simulink model "mainV02_28"  (R2016b)
settings: Solver=VariableStepAuto  StartTime=0.0  StopTime=Inf  FixedStep=0.001  MaxStep=0.2  RelTol=1e-2
undefined symbols (not defined in the file): checks, deltae_degrees, deltafl_degrees, deltafr_degrees, deltar_degrees, deltat_1, deltat_2, deltat_3, deltat_4, deltat_5, Earth, F, ft, groundReaction, initialValues, LD, Light, m, MIL, Newton, Raphson, s, sigbuilder_block, WGS84
libraries: aerolibutil x19, simulink x10, aerolibtransform2 x6, aerolibasang x4, aerolib6dofsys x4, aerolib6dof2 x4, aerolibwind2 x3, aerolibbdyn x3, aerolibconvert2 x3, aerolibconvert x2, vrlib x2, aerolibatmos2 x1
(part 5 of 5)

== system mainV02_28/LIBIS Plant/Propulsion/Variant_Motor_4/noMappedMotor_4/Propeller_4 ==
  RPM : Inport
  V_flight : Inport  Port=2
  airDensity : Inport  Port=3
  Constant : Constant  Value=5
  Constant1 : Constant  Value=3
  Constant2 : Constant  Value=4
  Constant3 : Constant  Value=2
  Cp Interpolation Using Prelookup : Interpolation_n-D  Table=LD.Propulsion.propeller4.Cp  ExtrapMethod=Clip  ValidIndexMayReachLast=on  InternalRulePriority=Speed
  Ct Interpolation Using Prelookup2 : Interpolation_n-D  Table=LD.Propulsion.propeller4.Ct  ExtrapMethod=Clip  ValidIndexMayReachLast=on  InternalRulePriority=Speed
  Diameter : Constant  Value=LD.Propulsion.propeller4.Diameter
  Gain : Gain  Gain=1/60
  Math Function{,1..3} (4 alike) : Math  Operator=pow  SaturateOnIntegerOverflow=on
  Prelookup4 : PreLookup  BreakpointsData=LD.Propulsion.propeller4.RPM  IndexSearchMethod=Evenly spaced points  UseLastBreakpoint=on
  Prelookup5 : PreLookup  BreakpointsData=LD.Propulsion.propeller4.V  UseLastBreakpoint=on
  Product : Product  Inputs=4
  Product1 : Product  Inputs=4
  RPM1 : InportShadow
  P_needed : Outport
  Thrust : Outport  Port=2
  wires:
  Diameter/1 -> Math Function2/1, Math Function/1  "D"
  Constant/1 -> Math Function/2  "5"
  Constant1/1 -> Math Function1/2  "3"
  Cp Interpolation Using Prelookup/1 -> Product/4  "Cp"
  Math Function1/1 -> Product/3  "n^3"
  Math Function/1 -> Product/2  "D^5"
  airDensity/1 -> Product/1, Product1/4  "airDensity"
  Product/1 -> P_needed/1  "Pneeded"
  Product1/1 -> Thrust/1  "Thrust"
  V_flight/1 -> Prelookup5/1  "V_flight"
  Constant2/1 -> Math Function2/2  "4"
  Math Function2/1 -> Product1/3  "D^4"
  Prelookup4/1 -> Cp Interpolation Using Prelookup/1, Ct Interpolation Using Prelookup2/1
  Prelookup4/2 -> Ct Interpolation Using Prelookup2/2, Cp Interpolation Using Prelookup/2
  Prelookup5/1 -> Cp Interpolation Using Prelookup/3, Ct Interpolation Using Prelookup2/3
  Prelookup5/2 -> Ct Interpolation Using Prelookup2/4, Cp Interpolation Using Prelookup/4
  Ct Interpolation Using Prelookup2/1 -> Product1/1  "Ct"
  Constant3/1 -> Math Function3/2  "2"
  Gain/1 -> Math Function1/1, Math Function3/1  "n_rev_s"
  Math Function3/1 -> Product1/2  "n^2"
  RPM1/1 -> Gain/1  "RPM"
  RPM/1 -> Prelookup4/1  "RPM"

== system mainV02_28/LIBIS Plant/Propulsion/Variant_Motor_4/noMappedMotor_4/Torque ==
  RPM : Inport
  Vflight : Inport  Port=2
  Constant : Constant  Value=1000
  Constant1 : Constant  Value=0
  RPM Prelookup : PreLookup  BreakpointsData=LD.Propulsion.propeller4.RPM(:,1)  IndexSearchMethod=Evenly spaced points  UseLastBreakpoint=on
  RPM1 : InportShadow
  Sum : Sum  Inputs=|-+
  Switch : Switch
  Torque Interpolation Using Prelookup : Interpolation_n-D  Table=LD.Propulsion.propeller4.Torque  ExtrapMethod=Clip  ValidIndexMayReachLast=on  InternalRulePriority=Speed
  Vflight Prelookup : PreLookup  BreakpointsData=LD.Propulsion.propeller4.V(1,:)  UseLastBreakpoint=on
  Torque : Outport
  wires:
  [k2] -> Torque Interpolation Using Prelookup/3
  RPM Prelookup/1 -> [k1]
  RPM Prelookup/2 -> [f1]
  [f1] -> Torque Interpolation Using Prelookup/2
  [k1] -> Torque Interpolation Using Prelookup/1
  [f2] -> Torque Interpolation Using Prelookup/4
  RPM/1 -> RPM Prelookup/1
  Vflight Prelookup/1 -> [k2]
  Vflight Prelookup/2 -> [f2]
  Vflight/1 -> Vflight Prelookup/1
  Torque Interpolation Using Prelookup/1 -> Switch/1  "Torque"
  Switch/1 -> Torque/1  "Torque"
  Sum/1 -> Switch/2
  Constant1/1 -> Switch/3
  Constant/1 -> Sum/1
  RPM1/1 -> Sum/2

== system mainV02_28/LIBIS Plant/Propulsion/Variant_Motor_5/mappedMotor_5/ESC_5 ==
  V_battery : Inport  Unit=V
  Throttle : Inport  Port=2  Unit=1
  Product : Product
  Product1 : Product
  eta_ESC : Constant  Value=LD.Propulsion.ESC5.eta
  V_ESC : Outport  Unit=V
  wires:
  eta_ESC/1 -> Product/2
  V_battery/1 -> Product/1
  Product/1 -> Product1/1
  Product1/1 -> V_ESC/1
  Throttle/1 -> Product1/2

== system mainV02_28/LIBIS Plant/Propulsion/Variant_Motor_5/mappedMotor_5/Motor and Propeller Coupling_5 ==
  Voltage : Inport
  Height : Inport  Port=2
  Vflight : Inport  Port=3
  Current Interpolation Using Prelookup : Interpolation_n-D  NumberOfTableDimensions=3  Table=LD.Propulsion.motor5.Current  ExtrapMethod=Clip  DiagnosticForOutOfRangeInput=Warning  ValidIndexMayReachLast=on  InternalRulePriority=Speed
      settings: InputPortMap=u0,u1,u2,u3,u4,u5
  Height Prelookup : PreLookup  BreakpointsData=LD.Propulsion.motor5.Height  IndexSearchMethod=Evenly spaced points  UseLastBreakpoint=on
  Power Interpolation Using Prelookup : Interpolation_n-D  NumberOfTableDimensions=3  Table=LD.Propulsion.motor5.Power  ExtrapMethod=Clip  DiagnosticForOutOfRangeInput=Warning  ValidIndexMayReachLast=on  InternalRulePriority=Speed
      settings: InputPortMap=u0,u1,u2,u3,u4,u5
  RPM Interpolation Using Prelookup : Interpolation_n-D  NumberOfTableDimensions=3  Table=LD.Propulsion.motor5.RPM  ExtrapMethod=Clip  DiagnosticForOutOfRangeInput=Warning  ValidIndexMayReachLast=on  InternalRulePriority=Speed
      settings: InputPortMap=u0,u1,u2,u3,u4,u5
  Thrust Interpolation Using Prelookup : Interpolation_n-D  NumberOfTableDimensions=3  Table=LD.Propulsion.motor5.Thrust  ExtrapMethod=Clip  DiagnosticForOutOfRangeInput=Warning  ValidIndexMayReachLast=on  InternalRulePriority=Speed
      settings: InputPortMap=u0,u1,u2,u3,u4,u5
  Vflight Prelookup : PreLookup  BreakpointsData=LD.Propulsion.motor5.Vflight  IndexSearchMethod=Evenly spaced points  UseLastBreakpoint=on
  Voltage Prelookup : PreLookup  BreakpointsData=LD.Propulsion.motor5.Voltage  IndexSearchMethod=Evenly spaced points  UseLastBreakpoint=on
  Thrust : Outport  PortDimensions=1
  Power : Outport  Port=2  PortDimensions=1
  Current : Outport  Port=3  PortDimensions=1
  RPM : Outport  Port=4  PortDimensions=1
  wires:
  Height/1 -> Height Prelookup/1
  Vflight/1 -> Vflight Prelookup/1
  RPM Interpolation Using Prelookup/1 -> RPM/1  "RPM"
  Power Interpolation Using Prelookup/1 -> Power/1  "Power"
  Thrust Interpolation Using Prelookup/1 -> Thrust/1  "Thrust"
  Current Interpolation Using Prelookup/1 -> Current/1  "Current"
  Voltage/1 -> Voltage Prelookup/1
  Voltage Prelookup/1 -> [k1]
  Voltage Prelookup/2 -> [f1]
  Height Prelookup/1 -> [k2]
  Height Prelookup/2 -> [f2]
  Vflight Prelookup/2 -> [f3]
  Vflight Prelookup/1 -> [k3]
  [k1] -> Thrust Interpolation Using Prelookup/1
  [k1] -> Power Interpolation Using Prelookup/1
  [k1] -> Current Interpolation Using Prelookup/1
  [k1] -> RPM Interpolation Using Prelookup/1
  [f1] -> Thrust Interpolation Using Prelookup/2
  [k2] -> Thrust Interpolation Using Prelookup/3
  [k2] -> Power Interpolation Using Prelookup/3
  [k2] -> Current Interpolation Using Prelookup/3
  [k2] -> RPM Interpolation Using Prelookup/3
  [k3] -> Thrust Interpolation Using Prelookup/5
  [k3] -> Power Interpolation Using Prelookup/5
  [k3] -> Current Interpolation Using Prelookup/5
  [k3] -> RPM Interpolation Using Prelookup/5
  [f1] -> Power Interpolation Using Prelookup/2
  [f1] -> Current Interpolation Using Prelookup/2
  [f1] -> RPM Interpolation Using Prelookup/2
  [f2] -> RPM Interpolation Using Prelookup/4
  [f2] -> Current Interpolation Using Prelookup/4
  [f2] -> Power Interpolation Using Prelookup/4
  [f2] -> Thrust Interpolation Using Prelookup/4
  [f3] -> RPM Interpolation Using Prelookup/6
  [f3] -> Current Interpolation Using Prelookup/6
  [f3] -> Power Interpolation Using Prelookup/6
  [f3] -> Thrust Interpolation Using Prelookup/6

== system mainV02_28/LIBIS Plant/Propulsion/Variant_Motor_5/mappedMotor_5/Torque ==
  RPM : Inport
  Vflight : Inport  Port=2
  Constant : Constant  Value=1000
  Constant1 : Constant  Value=0
  RPM Prelookup : PreLookup  BreakpointsData=LD.Propulsion.propeller5.RPM(:,1)  IndexSearchMethod=Evenly spaced points  UseLastBreakpoint=on
  RPM1 : InportShadow
  Sum : Sum  Inputs=|-+
  Switch : Switch
  Torque Interpolation Using Prelookup : Interpolation_n-D  Table=LD.Propulsion.propeller5.Torque  ExtrapMethod=Clip  ValidIndexMayReachLast=on  InternalRulePriority=Speed
  Vflight Prelookup : PreLookup  BreakpointsData=LD.Propulsion.propeller5.V(1,:)  UseLastBreakpoint=on
  Torque : Outport
  wires:
  [k2] -> Torque Interpolation Using Prelookup/3
  RPM Prelookup/1 -> [k1]
  RPM Prelookup/2 -> [f1]
  [f1] -> Torque Interpolation Using Prelookup/2
  [k1] -> Torque Interpolation Using Prelookup/1
  [f2] -> Torque Interpolation Using Prelookup/4
  RPM/1 -> RPM Prelookup/1
  Vflight Prelookup/1 -> [k2]
  Vflight Prelookup/2 -> [f2]
  Vflight/1 -> Vflight Prelookup/1
  Torque Interpolation Using Prelookup/1 -> Switch/1  "Torque"
  Switch/1 -> Torque/1  "Torque"
  Sum/1 -> Switch/2
  Constant1/1 -> Switch/3
  Constant/1 -> Sum/1
  RPM1/1 -> Sum/2

== system mainV02_28/LIBIS Plant/Propulsion/Variant_Motor_5/noMappedMotor_5/ESC_5 ==
  V_battery : Inport  Unit=V
  Throttle : Inport  Port=2  Unit=1
  Product : Product
  Product1 : Product
  eta_ESC : Constant  Value=LD.Propulsion.ESC5.eta
  V_ESC : Outport  Unit=V
  wires:
  eta_ESC/1 -> Product/2
  V_battery/1 -> Product/1
  Product/1 -> Product1/1
  Product1/1 -> V_ESC/1
  Throttle/1 -> Product1/2

== system mainV02_28/LIBIS Plant/Propulsion/Variant_Motor_5/noMappedMotor_5/Motor_5 ==
  V_ESC : Inport
  Im : Inport  Port=2
  ActiveMotor5 : Subsystem  VariantControl=Variants.Motor2~=0
  Constant : Constant  Value=LD.Propulsion.motor5.I0
  Constant1 : Constant  Value=LD.Propulsion.motor5.Rm
  Peje Switch : Switch  Criteria=u2 > Threshold
  Product : Product
  RPM Switch : Switch  Criteria=u2 > Threshold
  Sum : Sum  Inputs=|+-
  V_ESC1 : InportShadow
  noActiveMotor5 : Subsystem  VariantControl=Variants.Motor2==0
  RPM : Outport
  Peje : Outport  Port=2
  wires:
  V_ESC/1 -> noActiveMotor5/1(V_ESC), ActiveMotor5/1(V_ESC)
  Im/1 -> noActiveMotor5/2(Im), ActiveMotor5/2(Im)
  Sum/1 -> Peje Switch/2, RPM Switch/2
  Peje Switch/1 -> Peje/1
  RPM Switch/1 -> RPM/1
  ActiveMotor5/1(RPM) -> RPM Switch/1
  noActiveMotor5/1(RPM) -> RPM Switch/3
  noActiveMotor5/2(Peje) -> Peje Switch/3
  ActiveMotor5/2(Peje) -> Peje Switch/1
  V_ESC1/1 -> Sum/1
  Product/1 -> Sum/2
  Constant/1 -> Product/1
  Constant1/1 -> Product/2

== system mainV02_28/LIBIS Plant/Propulsion/Variant_Motor_5/noMappedMotor_5/Propeller_5 ==
  RPM : Inport
  V_flight : Inport  Port=2
  airDensity : Inport  Port=3
  Constant : Constant  Value=5
  Constant1 : Constant  Value=3
  Constant2 : Constant  Value=4
  Constant3 : Constant  Value=2
  Cp Interpolation Using Prelookup : Interpolation_n-D  Table=LD.Propulsion.propeller5.Cp  ExtrapMethod=Clip  ValidIndexMayReachLast=on  InternalRulePriority=Speed
  Ct Interpolation Using Prelookup2 : Interpolation_n-D  Table=LD.Propulsion.propeller5.Ct  ExtrapMethod=Clip  ValidIndexMayReachLast=on  InternalRulePriority=Speed
  Diameter : Constant  Value=LD.Propulsion.propeller5.Diameter
  Gain : Gain  Gain=1/60
  Math Function{,1..3} (4 alike) : Math  Operator=pow  SaturateOnIntegerOverflow=on
  Prelookup4 : PreLookup  BreakpointsData=LD.Propulsion.propeller5.RPM  IndexSearchMethod=Evenly spaced points  UseLastBreakpoint=on
  Prelookup5 : PreLookup  BreakpointsData=LD.Propulsion.propeller5.V  UseLastBreakpoint=on
  Product : Product  Inputs=4
  Product1 : Product  Inputs=4
  RPM1 : InportShadow
  P_needed : Outport
  Thrust : Outport  Port=2
  wires:
  Diameter/1 -> Math Function2/1, Math Function/1  "D"
  Constant/1 -> Math Function/2  "5"
  Constant1/1 -> Math Function1/2  "3"
  Cp Interpolation Using Prelookup/1 -> Product/4  "Cp"
  Math Function1/1 -> Product/3  "n^3"
  Math Function/1 -> Product/2  "D^5"
  airDensity/1 -> Product/1, Product1/4  "airDensity"
  Product/1 -> P_needed/1  "Pneeded"
  Product1/1 -> Thrust/1  "Thrust"
  V_flight/1 -> Prelookup5/1  "V_flight"
  Constant2/1 -> Math Function2/2  "4"
  Math Function2/1 -> Product1/3  "D^4"
  Prelookup4/1 -> Cp Interpolation Using Prelookup/1, Ct Interpolation Using Prelookup2/1
  Prelookup4/2 -> Ct Interpolation Using Prelookup2/2, Cp Interpolation Using Prelookup/2
  Prelookup5/1 -> Cp Interpolation Using Prelookup/3, Ct Interpolation Using Prelookup2/3
  Prelookup5/2 -> Cp Interpolation Using Prelookup/4, Ct Interpolation Using Prelookup2/4
  Ct Interpolation Using Prelookup2/1 -> Product1/1  "Ct"
  Constant3/1 -> Math Function3/2  "2"
  Gain/1 -> Math Function1/1, Math Function3/1  "n_rev_s"
  Math Function3/1 -> Product1/2  "n^2"
  RPM/1 -> Prelookup4/1  "RPM"
  RPM1/1 -> Gain/1  "RPM"

== system mainV02_28/LIBIS Plant/Propulsion/Variant_Motor_5/noMappedMotor_5/Torque ==
  RPM : Inport
  Vflight : Inport  Port=2
  Constant : Constant  Value=1000
  Constant1 : Constant  Value=0
  RPM Prelookup : PreLookup  BreakpointsData=LD.Propulsion.propeller5.RPM(:,1)  IndexSearchMethod=Evenly spaced points  UseLastBreakpoint=on
  RPM1 : InportShadow
  Sum : Sum  Inputs=|-+
  Switch : Switch
  Torque Interpolation Using Prelookup : Interpolation_n-D  Table=LD.Propulsion.propeller5.Torque  ExtrapMethod=Clip  ValidIndexMayReachLast=on  InternalRulePriority=Speed
  Vflight Prelookup : PreLookup  BreakpointsData=LD.Propulsion.propeller5.V(1,:)  UseLastBreakpoint=on
  Torque : Outport
  wires:
  [k2] -> Torque Interpolation Using Prelookup/3
  RPM Prelookup/1 -> [k1]
  RPM Prelookup/2 -> [f1]
  [f1] -> Torque Interpolation Using Prelookup/2
  [k1] -> Torque Interpolation Using Prelookup/1
  [f2] -> Torque Interpolation Using Prelookup/4
  RPM/1 -> RPM Prelookup/1
  Vflight Prelookup/1 -> [k2]
  Vflight Prelookup/2 -> [f2]
  Vflight/1 -> Vflight Prelookup/1
  Torque Interpolation Using Prelookup/1 -> Switch/1  "Torque"
  Switch/1 -> Torque/1  "Torque"
  Sum/1 -> Switch/2
  Constant1/1 -> Switch/3
  Constant/1 -> Sum/1
  RPM1/1 -> Sum/2

== system mainV02_28/LIBIS Plant/Propulsion/Variant_Motor_1/noMappedMotor_1/Motor_1/ActiveMotor1 ==
  V_ESC : Inport
  Im : Inport  Port=2
  Divide : Product  Inputs=*/*
  I0 : Constant  Value=LD.Propulsion.motor1.I0
  Kv : Constant  Value=LD.Propulsion.motor1.Kv
  Product : Product
  Product1 : Product
  Rm : Constant  Value=LD.Propulsion.motor1.Rm
  Sum : Sum  Inputs=+-
  Sum1 : Sum  Inputs=+-
  RPM : Outport
  Peje : Outport  Port=2
  wires:
  I0/1 -> Sum1/2  "I0"
  V_ESC/1 -> Sum/1
  Sum/1 -> Product/1  "Vm - Rm·Im"
  Im/1 -> Sum1/1, Product1/1
  Divide/1 -> Peje/1  "Peje"
  Kv/1 -> Divide/2, Product/2  "Kv"
  Product/1 -> RPM/1, Divide/1  "RPM"
  Rm/1 -> Product1/2  "Rm"
  Product1/1 -> Sum/2  "Rm·Im"
  Sum1/1 -> Divide/3  "Im-I0"

== system mainV02_28/LIBIS Plant/Propulsion/Variant_Motor_1/noMappedMotor_1/Motor_1/noActiveMotor1 ==
  V_ESC : Inport
  Im : Inport  Port=2
  Constant : Constant  Value=0
  Constant1 : Constant  Value=0
  Terminator : Terminator
  Terminator1 : Terminator
  RPM : Outport
  Peje : Outport  Port=2
  wires:
  V_ESC/1 -> Terminator/1
  Im/1 -> Terminator1/1
  Constant/1 -> RPM/1
  Constant1/1 -> Peje/1

== system mainV02_28/LIBIS Plant/Propulsion/Variant_Motor_2/noMappedMotor_2/Motor_2/ActiveMotor2 ==
  V_ESC : Inport
  Im : Inport  Port=2
  Divide : Product  Inputs=*/*
  I0 : Constant  Value=LD.Propulsion.motor2.I0
  Kv : Constant  Value=LD.Propulsion.motor2.Kv
  Product : Product
  Product1 : Product
  Rm : Constant  Value=LD.Propulsion.motor2.Rm
  Sum : Sum  Inputs=+-
  Sum1 : Sum  Inputs=+-
  RPM : Outport
  Peje : Outport  Port=2
  wires:
  I0/1 -> Sum1/2  "I0"
  V_ESC/1 -> Sum/1
  Sum/1 -> Product/1  "Vm - Rm·Im"
  Im/1 -> Sum1/1, Product1/1
  Divide/1 -> Peje/1  "Peje"
  Kv/1 -> Divide/2, Product/2  "Kv"
  Product/1 -> RPM/1, Divide/1  "RPM"
  Rm/1 -> Product1/2  "Rm"
  Product1/1 -> Sum/2  "Rm·Im"
  Sum1/1 -> Divide/3  "Im-I0"

== system mainV02_28/LIBIS Plant/Propulsion/Variant_Motor_2/noMappedMotor_2/Motor_2/noActiveMotor2 ==
  V_ESC : Inport
  Im : Inport  Port=2
  Constant : Constant  Value=0
  Constant1 : Constant  Value=0
  Terminator : Terminator
  Terminator1 : Terminator
  RPM : Outport
  Peje : Outport  Port=2
  wires:
  V_ESC/1 -> Terminator/1
  Im/1 -> Terminator1/1
  Constant/1 -> RPM/1
  Constant1/1 -> Peje/1

== system mainV02_28/LIBIS Plant/Propulsion/Variant_Motor_3/noMappedMotor_3/Motor_3/ActiveMotor3 ==
  V_ESC : Inport
  Im : Inport  Port=2
  Divide : Product  Inputs=*/*
  I0 : Constant  Value=LD.Propulsion.motor3.I0
  Kv : Constant  Value=LD.Propulsion.motor3.Kv
  Product : Product
  Product1 : Product
  Rm : Constant  Value=LD.Propulsion.motor3.Rm
  Sum : Sum  Inputs=+-
  Sum1 : Sum  Inputs=+-
  RPM : Outport
  Peje : Outport  Port=2
  wires:
  I0/1 -> Sum1/2  "I0"
  V_ESC/1 -> Sum/1
  Sum/1 -> Product/1  "Vm - Rm·Im"
  Im/1 -> Sum1/1, Product1/1
  Divide/1 -> Peje/1  "Peje"
  Kv/1 -> Divide/2, Product/2  "Kv"
  Product/1 -> RPM/1, Divide/1  "RPM"
  Rm/1 -> Product1/2  "Rm"
  Product1/1 -> Sum/2  "Rm·Im"
  Sum1/1 -> Divide/3  "Im-I0"

== system mainV02_28/LIBIS Plant/Propulsion/Variant_Motor_3/noMappedMotor_3/Motor_3/noActiveMotor3 ==
  V_ESC : Inport
  Im : Inport  Port=2
  Constant : Constant  Value=0
  Constant1 : Constant  Value=0
  Terminator : Terminator
  Terminator1 : Terminator
  RPM : Outport
  Peje : Outport  Port=2
  wires:
  V_ESC/1 -> Terminator/1
  Im/1 -> Terminator1/1
  Constant/1 -> RPM/1
  Constant1/1 -> Peje/1

== system mainV02_28/LIBIS Plant/Propulsion/Variant_Motor_4/noMappedMotor_4/Motor_4/ActiveMotor4 ==
  V_ESC : Inport
  Im : Inport  Port=2
  Divide : Product  Inputs=*/*
  I0 : Constant  Value=LD.Propulsion.motor4.I0
  Kv : Constant  Value=LD.Propulsion.motor4.Kv
  Product : Product
  Product1 : Product
  Rm : Constant  Value=LD.Propulsion.motor4.Rm
  Sum : Sum  Inputs=+-
  Sum1 : Sum  Inputs=+-
  RPM : Outport
  Peje : Outport  Port=2
  wires:
  I0/1 -> Sum1/2  "I0"
  V_ESC/1 -> Sum/1
  Sum/1 -> Product/1  "Vm - Rm·Im"
  Im/1 -> Sum1/1, Product1/1
  Divide/1 -> Peje/1  "Peje"
  Kv/1 -> Divide/2, Product/2  "Kv"
  Product/1 -> RPM/1, Divide/1  "RPM"
  Rm/1 -> Product1/2  "Rm"
  Product1/1 -> Sum/2  "Rm·Im"
  Sum1/1 -> Divide/3  "Im-I0"

== system mainV02_28/LIBIS Plant/Propulsion/Variant_Motor_4/noMappedMotor_4/Motor_4/noActiveMotor4 ==
  V_ESC : Inport
  Im : Inport  Port=2
  Constant : Constant  Value=0
  Constant1 : Constant  Value=0
  Terminator : Terminator
  Terminator1 : Terminator
  RPM : Outport
  Peje : Outport  Port=2
  wires:
  V_ESC/1 -> Terminator/1
  Im/1 -> Terminator1/1
  Constant/1 -> RPM/1
  Constant1/1 -> Peje/1

== system mainV02_28/LIBIS Plant/Propulsion/Variant_Motor_5/noMappedMotor_5/Motor_5/ActiveMotor5 ==
  V_ESC : Inport
  Im : Inport  Port=2
  Divide : Product  Inputs=*/*
  I0 : Constant  Value=LD.Propulsion.motor5.I0
  Kv : Constant  Value=LD.Propulsion.motor5.Kv
  Product : Product
  Product1 : Product
  Rm : Constant  Value=LD.Propulsion.motor5.Rm
  Sum : Sum  Inputs=+-
  Sum1 : Sum  Inputs=+-
  RPM : Outport
  Peje : Outport  Port=2
  wires:
  I0/1 -> Sum1/2  "I0"
  V_ESC/1 -> Sum/1
  Sum/1 -> Product/1  "Vm - Rm·Im"
  Im/1 -> Sum1/1, Product1/1
  Divide/1 -> Peje/1  "Peje"
  Kv/1 -> Divide/2, Product/2  "Kv"
  Product/1 -> RPM/1, Divide/1  "RPM"
  Rm/1 -> Product1/2  "Rm"
  Product1/1 -> Sum/2  "Rm·Im"
  Sum1/1 -> Divide/3  "Im-I0"

== system mainV02_28/LIBIS Plant/Propulsion/Variant_Motor_5/noMappedMotor_5/Motor_5/noActiveMotor5 ==
  V_ESC : Inport
  Im : Inport  Port=2
  Constant : Constant  Value=0
  Constant1 : Constant  Value=0
  Terminator : Terminator
  Terminator1 : Terminator
  RPM : Outport
  Peje : Outport  Port=2
  wires:
  V_ESC/1 -> Terminator/1
  Im/1 -> Terminator1/1
  Constant/1 -> RPM/1
  Constant1/1 -> Peje/1
